simulink subsystem "Subsystem_Sensores"  (R2023b)
settings: Solver=VariableStepAuto  StartTime=0.0  StopTime=10.0  RelTol=1e-3
libraries: arduinolib x2
settings Model: Creator=Alberto  LastModifiedBy=Alberto

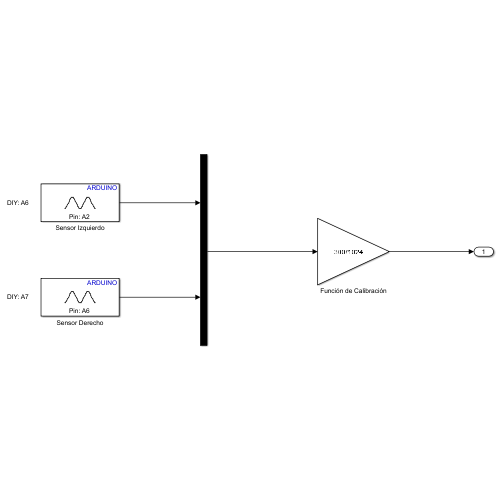
[thumbnail: Simulink's stored preview of the top-level diagram]
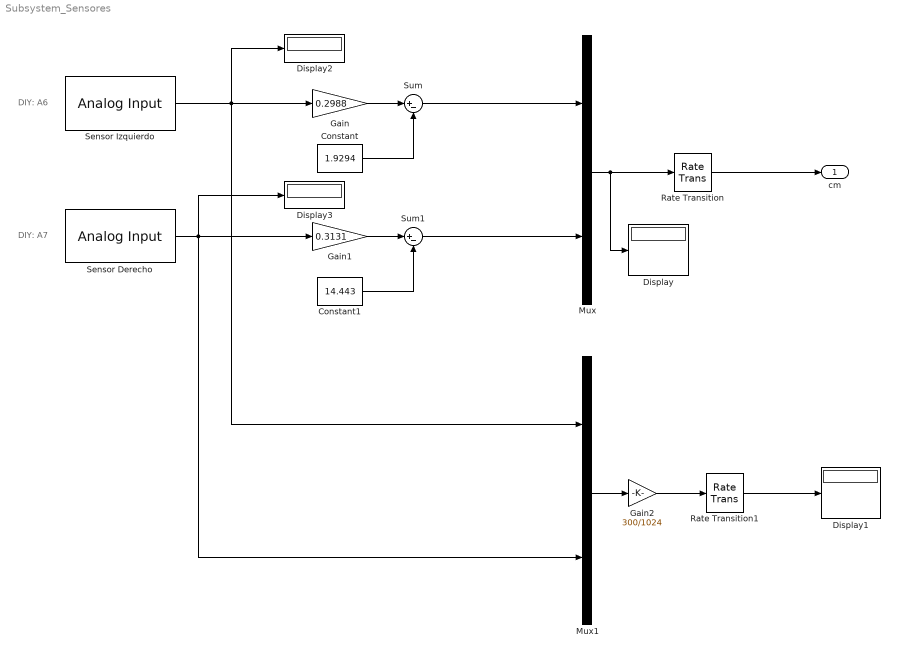
== system Subsystem_Sensores ==
  note: DIY: A7
  note: DIY: A6
  Constant : Constant  Value=1.9294
  Constant1 : Constant  Value=14.443
  Display{,1..3} (4 alike) : Display
  Gain : Gain  Gain=0.2988
  Gain1 : Gain  Gain=0.3131
  Gain2 : Gain  Gain=300/1024
  Mux : Mux  Inputs=2
  Mux1 : Mux  Inputs=2
  Rate Transition : RateTransition
  Rate Transition1 : RateTransition
  Sensor Derecho : arduinolib/Analog Input  pinNumber=7  ReadResultsOnly=off  ConversionTriggerSource=Software  ExternalTriggerType=uint32( 0 )  OutputDataType=uint16  EnableConversionCompleteNotify=off  EnableOuputStatus=off  SampleTime=0.05  blockPlatform=arduino
  Sensor Izquierdo : arduinolib/Analog Input  pinNumber=6  ReadResultsOnly=off  ConversionTriggerSource=Software  ExternalTriggerType=uint32( 0 )  OutputDataType=uint16  EnableConversionCompleteNotify=off  EnableOuputStatus=off  SampleTime=0.05  blockPlatform=arduino
  Sum : Sum  Inputs=|+-
  Sum1 : Sum  Inputs=|+-
  cm : Outport
  wires:
  Mux/1 -> Rate Transition/1, Display/1
  Sensor Derecho/1 -> Gain1/1, Mux1/2, Display3/1
  Sensor Izquierdo/1 -> Gain/1, Display2/1, Mux1/1
  Gain/1 -> Sum/1
  Sum/1 -> Mux/1
  Gain1/1 -> Sum1/1
  Sum1/1 -> Mux/2
  Constant/1 -> Sum/2
  Constant1/1 -> Sum1/2
  Mux1/1 -> Gain2/1
  Gain2/1 -> Rate Transition1/1
  Rate Transition/1 -> cm/1
  Rate Transition1/1 -> Display1/1
